simulink model "FlightSim"  (R2019b)
settings: Solver=VariableStepAuto  StartTime=0.0  StopTime=185  RelTol=1e-3
values from neighbouring files (symbols this model uses):
  Thrust = xlsread('C:\Users\jpraj\Desktop\FinalSim\AscentMotor.csv','B2:B253')    [FlightSimulation.m]
  thrust = xlsread('C:\Users\jpraj\Desktop\FinalSim\DescentMotor.csv','B2:B795')    [FlightSimulation.m]
  Time = xlsread('C:\Users\jpraj\Desktop\FinalSim\AscentMotor.csv','A2:A253')    [FlightSimulation.m]
  time = xlsread('C:\Users\jpraj\Desktop\FinalSim\DescentMotor.csv','A2:A795')    [FlightSimulation.m]
libraries: aerolibatmos2 x3, simulink x1
settings Model: Creator=DHRUVAN MS  LastModifiedBy=jpraj
settings DataIOCC: ReturnWorkspaceOutputs=off
settings DebuggingCC: ArithmeticOperatorsInVariantConditions=warning
settings SFSimCC: SimUseLocalCustomCode=off  CustomCodeUndefinedFunction=UseInterfaceOnly
settings RTWCC: RTWUseLocalCustomCode=off
settings CodeAppCC: StateflowObjectComments=on

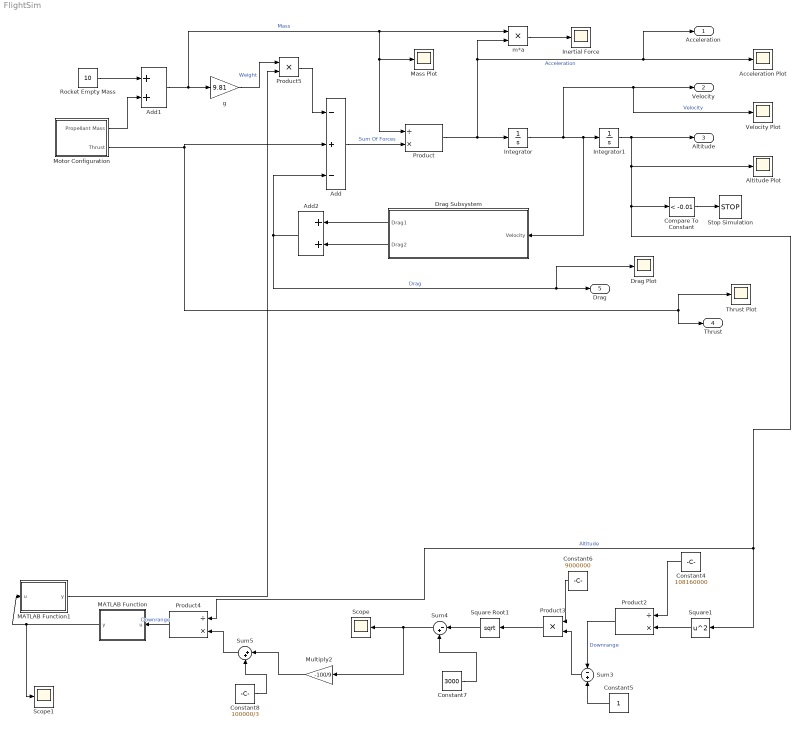
== system FlightSim ==
  Acceleration Plot : Scope
  Add : Sum  Inputs=-+-
  Add1 : Sum
  Add2 : Sum
  Altitude Plot : Scope
  Compare To Constant : simulink/Logic and Bit Operations/Compare To Constant  relop=<  const=-0.01  OutDataTypeStr=boolean
  Constant4 : Constant  Value=108160000
  Constant5 : Constant
  Constant6 : Constant  Value=9000000
  Constant7 : Constant  Value=3000
  Constant8 : Constant  Value=100000/3
  Drag Plot : Scope
  Drag Subsystem : Subsystem
  Inertial Force : Scope
  Integrator : Integrator
  Integrator1 : Integrator
  MATLAB Function : MATLAB Function  TreatAsAtomicUnit=on
  MATLAB Function1 : MATLAB Function  TreatAsAtomicUnit=on
  Mass Plot : Scope
  Motor Configuration : Subsystem  TreatAsAtomicUnit=on
  Multiply2 : Gain  Gain=-100/9
  Product : Product  Inputs=/*
  Product2 : Product  Inputs=/*
  Product3 : Product
  Product4 : Product  Inputs=/*
  Product5 : Product
  Rocket Empty Mass : Constant  Value=10
  Scope : Scope
  Scope1 : Scope
  Square Root1 : Sqrt  SaturateOnIntegerOverflow=on
  Square1 : Math  Operator=square  SignedPower=off  SaturateOnIntegerOverflow=on
  Stop Simulation : Stop
  Sum3 : Sum  Inputs=-+
  Sum4 : Sum  Inputs=|-+
  Sum5 : Sum  Inputs=|++
  Thrust Plot : Scope
  Velocity Plot : Scope
  g : Gain  Gain=9.81
  m*a : Product
  Acceleration : Outport
  Velocity : Outport  Port=2
  Altitude : Outport  Port=3
  Thrust : Outport  Port=4
  Drag : Outport  Port=5
  wires:
  Rocket Empty Mass/1 -> Add1/1
  Add1/1 -> g/1, Mass Plot/1, Product/1, m*a/1  "Mass"
  Add/1 -> Product/2  "Sum Of Forces"
  Integrator/1 -> Drag Subsystem/1(Velocity), Integrator1/1, Velocity Plot/1, Velocity/1  "Velocity"
  Integrator1/1 -> Compare To Constant/1, Square1/1, Product4/1, Altitude Plot/1, Altitude/1  "Altitude"
  Compare To Constant/1 -> Stop Simulation/1
  Product/1 -> Integrator/1, m*a/2, Acceleration/1, Acceleration Plot/1  "Acceleration"
  m*a/1 -> Inertial Force/1
  Motor Configuration/2(Thrust) -> Add/2, Thrust/1, Thrust Plot/1
  Motor Configuration/1(Propellant Mass) -> Add1/2
  Add2/1 -> Add/3, Drag/1, Drag Plot/1  "Drag"
  Drag Subsystem/1(Drag1) -> Add2/1
  Drag Subsystem/2(Drag2) -> Add2/2
  Square1/1 -> Product2/2
  Constant4/1 -> Product2/1
  Product2/1 -> Sum3/1  "Downrange"
  Constant5/1 -> Sum3/2
  Sum3/1 -> Product3/2
  Constant6/1 -> Product3/1
  Product3/1 -> Square Root1/1
  Square Root1/1 -> Sum4/1
  Constant7/1 -> Sum4/2
  Sum4/1 -> Multiply2/1, Scope/1
  Multiply2/1 -> Sum5/1
  Constant8/1 -> Sum5/2
  Sum5/1 -> Product4/2
  Product4/1 -> MATLAB Function/1(u)  "Downrange"
  g/1 -> Product5/1  "Weight"
  Product5/1 -> Add/1
  MATLAB Function/1(y) -> Scope1/1, MATLAB Function1/1(u)
  MATLAB Function1/1(y) -> Product5/2

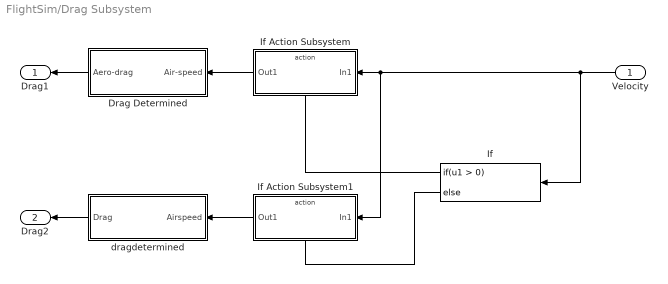
== system FlightSim/Drag Subsystem ==
  Velocity : Inport
  Drag Determined : Subsystem
  If : If
  If Action Subsystem : Subsystem  TreatAsAtomicUnit=on
  If Action Subsystem1 : Subsystem  TreatAsAtomicUnit=on
  dragdetermined : Subsystem
  Drag1 : Outport
  Drag2 : Outport  Port=2
  wires:
  If Action Subsystem1/1(Out1) -> dragdetermined/1(Airspeed)
  dragdetermined/1(Drag) -> Drag2/1
  If Action Subsystem/1(Out1) -> Drag Determined/1(Air-speed)
  Velocity/1 -> If/1, If Action Subsystem1/1(In1), If Action Subsystem/1(In1)
  Drag Determined/1(Aero-drag) -> Drag1/1
  If/2 -> If Action Subsystem1/Action
  If/1 -> If Action Subsystem/Action

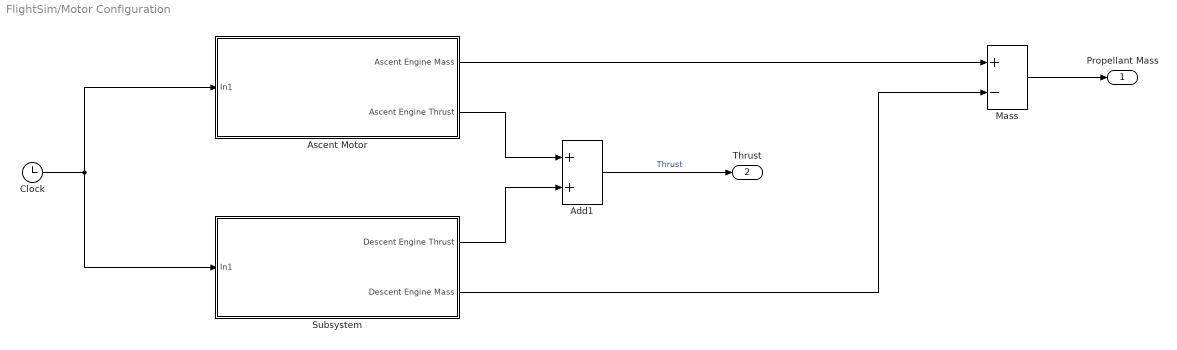
== system FlightSim/Motor Configuration ==
  Add1 : Sum
  "Ascent Motor " : Subsystem
  Clock : Clock
      settings: Decimation=100
  Mass : Sum  Inputs=+-
  Subsystem : Subsystem
  Propellant Mass : Outport
  Thrust : Outport  Port=2
  wires:
  Clock/1 -> Subsystem/1(In1), "Ascent Motor "/1(In1)
  Add1/1 -> Thrust/1  "Thrust"
  "Ascent Motor "/2(Ascent Engine Thrust) -> Add1/1
  Subsystem/1("Descent Engine Thrust ") -> Add1/2
  "Ascent Motor "/1(Ascent Engine Mass) -> Mass/1
  Subsystem/2(Descent Engine Mass) -> Mass/2
  Mass/1 -> Propellant Mass/1

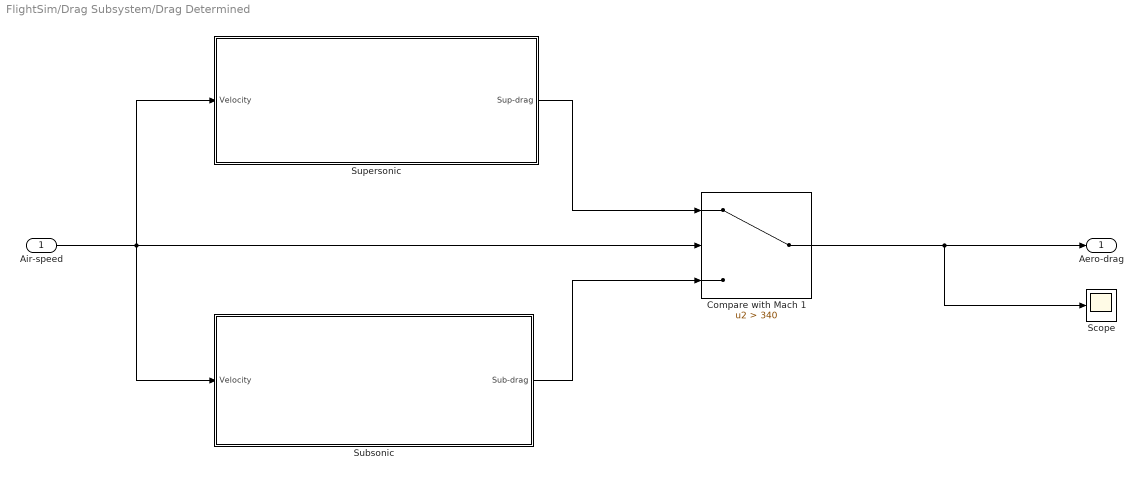
== system FlightSim/Drag Subsystem/Drag Determined ==
  Air-speed : Inport
  Compare with Mach 1 : Switch  Criteria=u2 > Threshold  Threshold=340
  Scope : Scope
  Subsonic : Subsystem
  Supersonic : Subsystem
  Aero-drag : Outport
  wires:
  Compare with Mach 1/1 -> Aero-drag/1, Scope/1
  Air-speed/1 -> Supersonic/1(Velocity), Compare with Mach 1/2, Subsonic/1(Velocity)
  Supersonic/1(Sup-drag) -> Compare with Mach 1/1
  Subsonic/1(Sub-drag) -> Compare with Mach 1/3

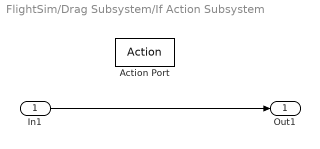
== system FlightSim/Drag Subsystem/If Action Subsystem ==
  In1 : Inport
  Action Port : ActionPort  ActionPortLabel=if(u1 > 0)
  Out1 : Outport
  wires:
  In1/1 -> Out1/1

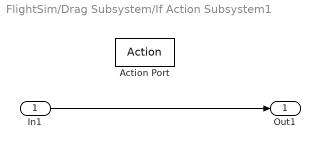
== system FlightSim/Drag Subsystem/If Action Subsystem1 ==
  In1 : Inport
  Action Port : ActionPort  ActionPortLabel=else
  Out1 : Outport
  wires:
  In1/1 -> Out1/1

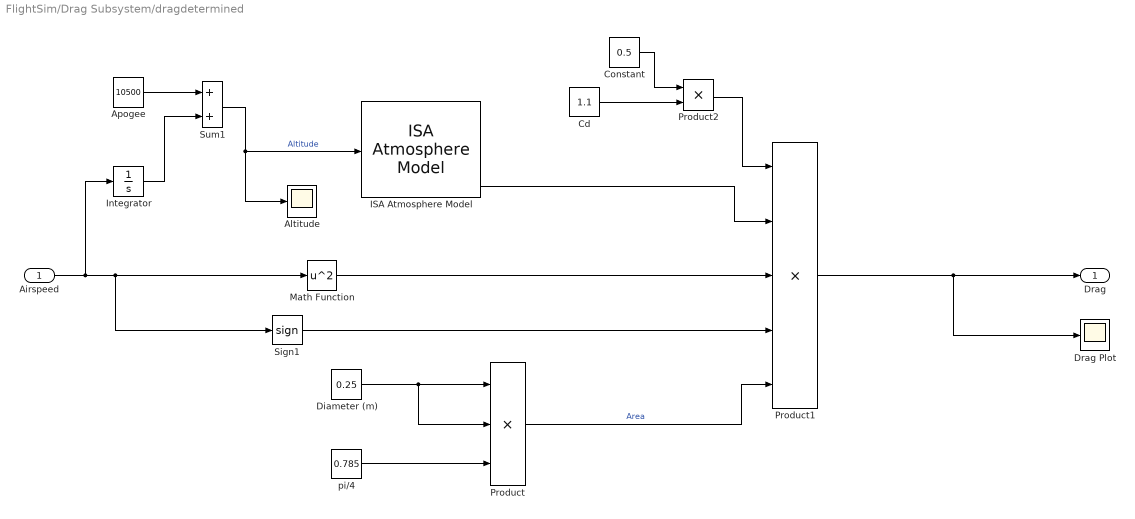
== system FlightSim/Drag Subsystem/dragdetermined ==
  Airspeed : Inport
  "Altitude " : Scope
  Apogee : Constant  Value=10500
  Cd : Constant  Value=1.1
  Constant : Constant  Value=0.5
  Diameter (m) : Constant  Value=0.25
  "Drag Plot " : Scope
  ISA Atmosphere Model : aerolibatmos2/ISA Atmosphere Model  custom=off  g=9.80665  gamma=1.4  R=287.0531  L=0.0065  h_trop=11000  h_strat=20000  rho0=1.225  P0=101325  T0=288.15  h0=0
      settings: SourceProductName=Aerospace Blockset
  Integrator : Integrator
  Math Function : Math  Operator=square  SaturateOnIntegerOverflow=on
  Product : Product  Inputs=3
  Product1 : Product  Inputs=5
  Product2 : Product
  Sign1 : Signum
  Sum1 : Sum
  pi/4 : Constant  Value=0.785
  Drag : Outport
  wires:
  pi/4/1 -> Product/3
  Diameter (m)/1 -> Product/2, Product/1
  Math Function/1 -> Product1/3
  Product2/1 -> Product1/1
  Constant/1 -> Product2/1
  Airspeed/1 -> Sign1/1, Math Function/1, Integrator/1
  Product1/1 -> "Drag Plot "/1, Drag/1
  ISA Atmosphere Model/4 -> Product1/2
  Cd/1 -> Product2/2
  Product/1 -> Product1/5  "Area"
  Sign1/1 -> Product1/4
  Integrator/1 -> Sum1/2
  Apogee/1 -> Sum1/1
  Sum1/1 -> "Altitude "/1, ISA Atmosphere Model/1  "Altitude"

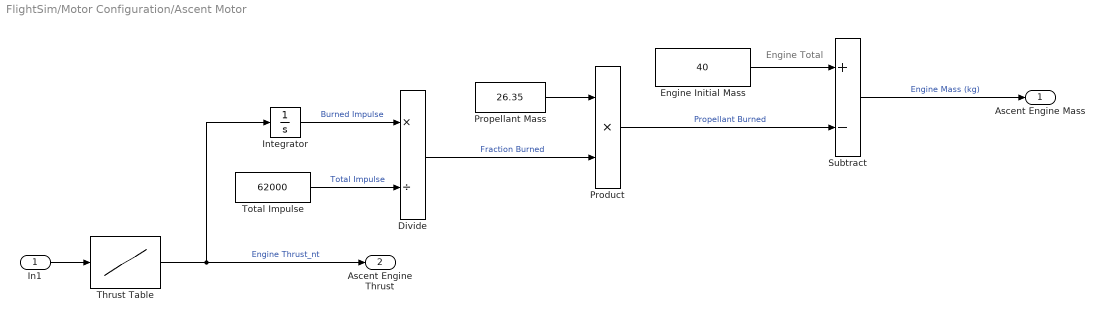
== system FlightSim/Motor Configuration/Ascent Motor  ==
  note: Engine Total
  In1 : Inport
  Divide : Product  Inputs=*/
  Engine Initial Mass : Constant  Value=40
  Integrator : Integrator
  Product : Product
  Propellant Mass : Constant  Value=26.35
  Subtract : Sum  Inputs=+-
  Thrust Table : Lookup_n-D  NumberOfTableDimensions=1  BreakpointsForDimension1=Time  Table=Thrust  InternalRulePriority=Speed  RndMeth=Simplest
  Total Impulse : Constant  Value=62000
  Ascent Engine Mass : Outport
  Ascent Engine Thrust : Outport  Port=2
  wires:
  Subtract/1 -> Ascent Engine Mass/1  "Engine Mass (kg)"
  Divide/1 -> Product/2  "Fraction Burned"
  Thrust Table/1 -> Ascent Engine Thrust/1, Integrator/1  "Engine Thrust_nt"
  Propellant Mass/1 -> Product/1
  Total Impulse/1 -> Divide/2  "Total Impulse"
  Integrator/1 -> Divide/1  "Burned Impulse"
  In1/1 -> Thrust Table/1
  Engine Initial Mass/1 -> Subtract/1
  Product/1 -> Subtract/2  "Propellant Burned"

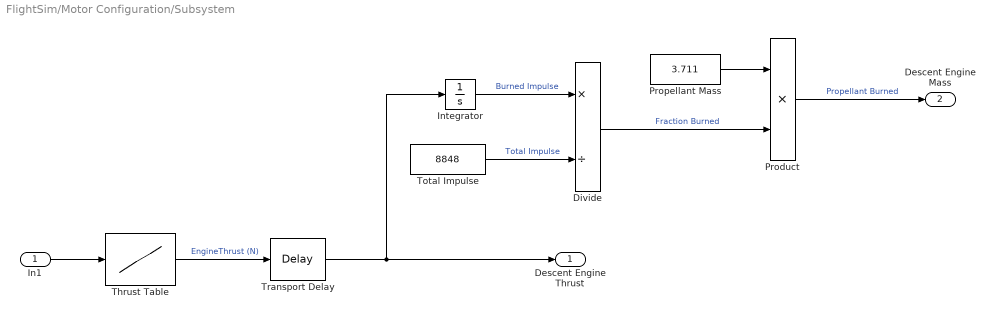
== system FlightSim/Motor Configuration/Subsystem ==
  In1 : Inport
  Divide : Product  Inputs=*/
  Integrator : Integrator
  Product : Product
  Propellant Mass : Constant  Value=3.711
  Thrust Table : Lookup_n-D  NumberOfTableDimensions=1  BreakpointsForDimension1=time  IndexSearchMethod=Linear search  Table=thrust  ExtrapMethod=Clip  InternalRulePriority=Speed  RndMeth=Simplest  InputSameDT=on
  Total Impulse : Constant  Value=8848
  Transport Delay : TransportDelay  DelayTime=129.75
  "Descent Engine Thrust " : Outport
  Descent Engine Mass : Outport  Port=2
  wires:
  Integrator/1 -> Divide/1  "Burned Impulse"
  Thrust Table/1 -> Transport Delay/1  "EngineThrust (N)"
  Transport Delay/1 -> "Descent Engine Thrust "/1, Integrator/1
  Total Impulse/1 -> Divide/2  "Total Impulse"
  Propellant Mass/1 -> Product/1
  Divide/1 -> Product/2  "Fraction Burned"
  In1/1 -> Thrust Table/1
  Product/1 -> Descent Engine Mass/1  "Propellant Burned"

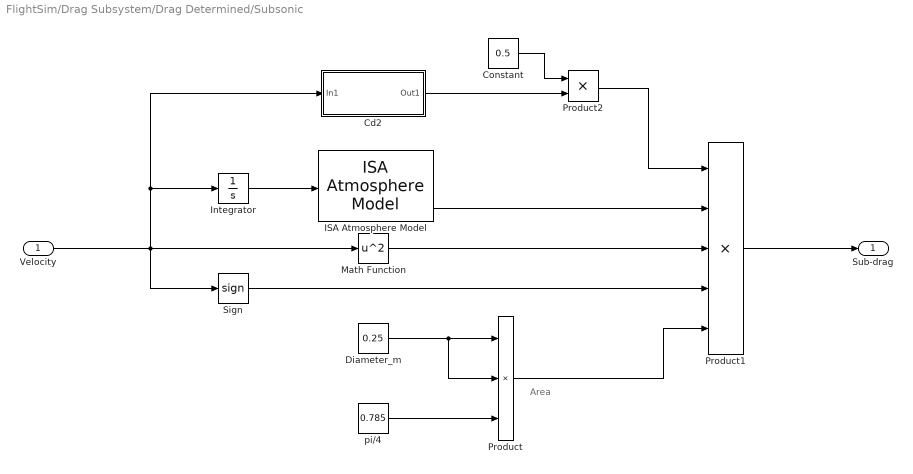
== system FlightSim/Drag Subsystem/Drag Determined/Subsonic ==
  note: Area
  Velocity : Inport
  Cd2 : Subsystem  TreatAsAtomicUnit=on
  Constant : Constant  Value=0.5
  Diameter_m : Constant  Value=0.25
  ISA Atmosphere Model : aerolibatmos2/ISA Atmosphere Model  custom=off  g=9.80665  gamma=1.4  R=287.0531  L=0.0065  h_trop=11000  h_strat=20000  rho0=1.225  P0=101325  T0=288.15  h0=0
      settings: SourceProductName=Aerospace Blockset
  Integrator : Integrator
  Math Function : Math  Operator=square  SaturateOnIntegerOverflow=on
  Product : Product  Inputs=3
  Product1 : Product  Inputs=5
  Product2 : Product
  Sign : Signum
  pi/4 : Constant  Value=0.785
  Sub-drag : Outport
  wires:
  ISA Atmosphere Model/4 -> Product1/2
  Constant/1 -> Product2/1
  Integrator/1 -> ISA Atmosphere Model/1
  Velocity/1 -> Sign/1, Cd2/1(In1), Integrator/1, Math Function/1
  Sign/1 -> Product1/4
  Product/1 -> Product1/5
  Diameter_m/1 -> Product/2, Product/1
  pi/4/1 -> Product/3
  Product2/1 -> Product1/1
  Math Function/1 -> Product1/3
  Cd2/1(Out1) -> Product2/2
  Product1/1 -> Sub-drag/1

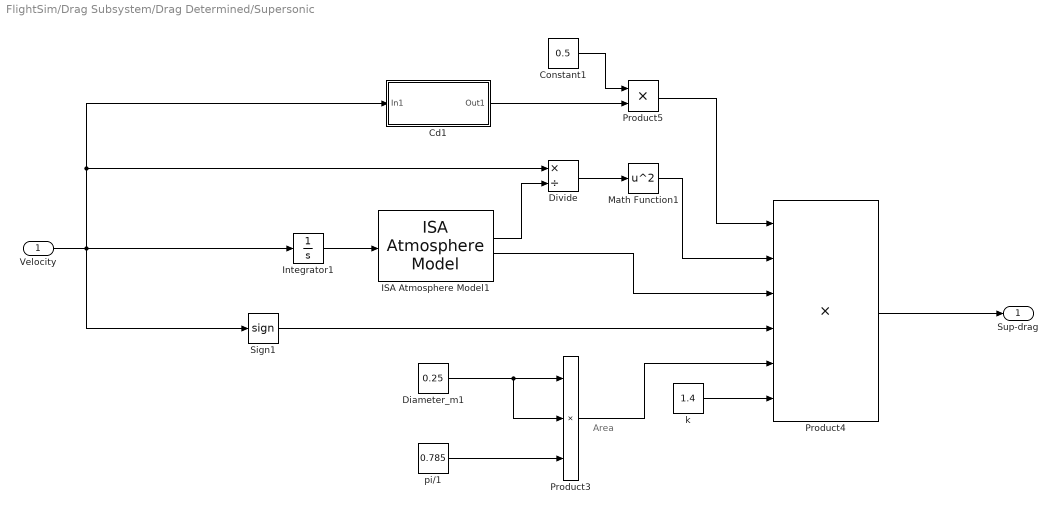
== system FlightSim/Drag Subsystem/Drag Determined/Supersonic ==
  note: Area
  Velocity : Inport
  Cd1 : Subsystem  TreatAsAtomicUnit=on
  Constant1 : Constant  Value=0.5
  Diameter_m1 : Constant  Value=0.25
  Divide : Product  Inputs=*/
  ISA Atmosphere Model1 : aerolibatmos2/ISA Atmosphere Model  custom=off  g=9.80665  gamma=1.4  R=287.0531  L=0.0065  h_trop=11000  h_strat=20000  rho0=1.225  P0=101325  T0=288.15  h0=0
      settings: SourceProductName=Aerospace Blockset
  Integrator1 : Integrator
  Math Function1 : Math  Operator=square  SaturateOnIntegerOverflow=on
  Product3 : Product  Inputs=3
  Product4 : Product  Inputs=6
  Product5 : Product
  Sign1 : Signum
  k : Constant  Value=1.4
  pi/1 : Constant  Value=0.785
  Sup-drag : Outport
  wires:
  Divide/1 -> Math Function1/1
  Cd1/1(Out1) -> Product5/2
  Diameter_m1/1 -> Product3/2, Product3/1
  Velocity/1 -> Cd1/1(In1), Divide/1, Sign1/1, Integrator1/1
  pi/1/1 -> Product3/3
  Product5/1 -> Product4/1
  Product3/1 -> Product4/5
  Constant1/1 -> Product5/1
  Sign1/1 -> Product4/4
  k/1 -> Product4/6
  ISA Atmosphere Model1/2 -> Divide/2
  Integrator1/1 -> ISA Atmosphere Model1/1
  Product4/1 -> Sup-drag/1
  ISA Atmosphere Model1/3 -> Product4/3
  Math Function1/1 -> Product4/2

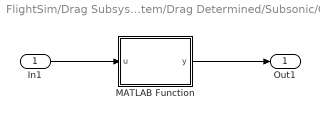
== system FlightSim/Drag Subsystem/Drag Determined/Subsonic/Cd2 ==
  In1 : Inport
  MATLAB Function : MATLAB Function  TreatAsAtomicUnit=on
  Out1 : Outport
  wires:
  In1/1 -> MATLAB Function/1(u)
  MATLAB Function/1(y) -> Out1/1

== system FlightSim/Drag Subsystem/Drag Determined/Supersonic/Cd1 ==
  In1 : Inport
  MATLAB Function : MATLAB Function  TreatAsAtomicUnit=on
  Out1 : Outport
  wires:
  In1/1 -> MATLAB Function/1(u)
  MATLAB Function/1(y) -> Out1/1

== matlab function FlightSim/Drag Subsystem/Drag Determined/Supersonic/Cd1/MATLAB Function ==
  data: u input; y output
function y = fcn(u)
M=u/340;
p=0;
coder.extrinsic('xlsread');
A = xlsread('C:\Users\jpraj\Desktop\FinalSim\Cd.xlsx','B2:B201');
y=0;
for i=0:0.01:2
    j=0+i;
    k=0.01+i;
    if (j<M)&&(M<=k)
        n=1+p;
        y=A(n);
    break
    else
        p=p+1;
    end
end

== matlab function FlightSim/Drag Subsystem/Drag Determined/Subsonic/Cd2/MATLAB Function ==
  data: u input; y output
function y = fcn(u)
M=u/340;
p=0;
coder.extrinsic('xlsread');
A = xlsread('C:\Users\jpraj\Desktop\FinalSim\Cd.xlsx','B2:B201');
y=0;
for i=0:0.01:2
    j=0+i;
    k=0.01+i;
    if (j<M)&&(M<=k)
        n=1+p;
        y=A(n);
    break
    else
        p=p+1;
    end
end

== matlab function FlightSim/MATLAB Function ==
  data: u input; y output
function y = fcn(u)
h=atan(u);

y = h;

== matlab function FlightSim/MATLAB Function1 ==
  data: u input; y output
function y = fcn(u)
i=sin(u);
y = i;
